simulink model "Loopshaping"  (R2023b)
settings: Solver=VariableStepAuto  StartTime=0.0  StopTime=10.0  RelTol=1e-3
settings Model: Creator=ADMIN  LastModifiedBy=ADMIN

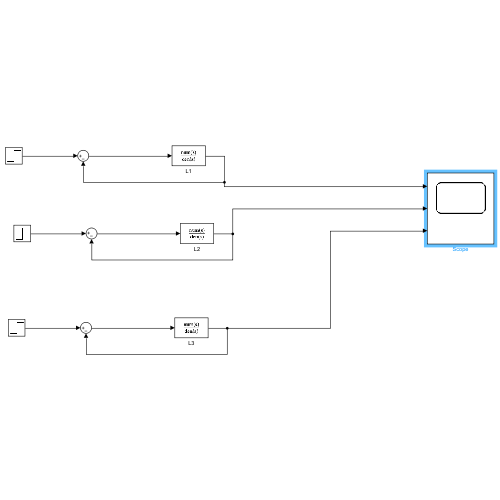
[thumbnail: Simulink's stored preview of the top-level diagram]
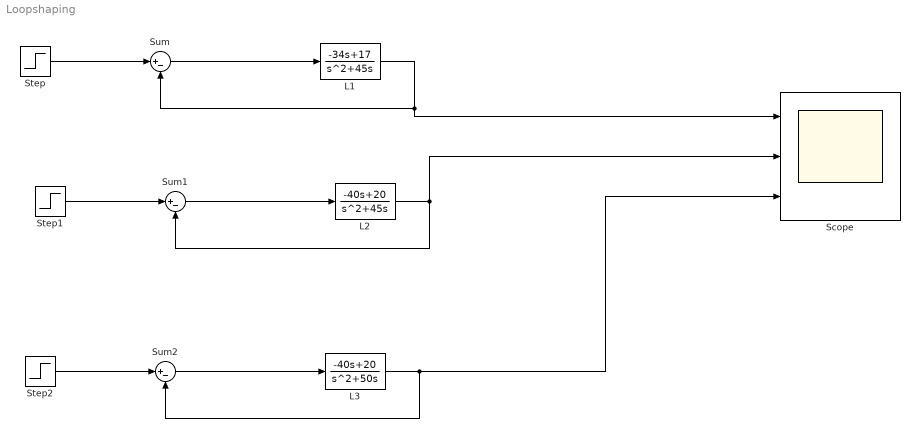
== system Loopshaping ==
  L1 : TransferFcn  Numerator="[0   -34    17]"  Denominator="[1    45     0]"
  L2 : TransferFcn  Numerator=|  Denominator="[1    45     0]"
      | [0   -40    20
      | ]
  L3 : TransferFcn  Numerator=|  Denominator="[1    50     0]"
      | [0   -40    20
      | ]
  Scope : Scope  NumInputPorts=3
  Step : Step  SampleTime=0
  Step1 : Step  SampleTime=0
  Step2 : Step  SampleTime=0
  Sum : Sum  Inputs=|+-
  Sum1 : Sum  Inputs=|+-
  Sum2 : Sum  Inputs=|+-
  wires:
  Step/1 -> Sum/1
  L1/1 -> Scope/1, Sum/2
  Step1/1 -> Sum1/1
  L2/1 -> Scope/2, Sum1/2
  Step2/1 -> Sum2/1
  L3/1 -> Scope/3, Sum2/2
  Sum/1 -> L1/1
  Sum1/1 -> L2/1
  Sum2/1 -> L3/1
